simulink model "Quad_Nonlinear_Pitch_Model"  (R2020a)
settings: Solver=ode3  StartTime=0.0  StopTime=10  FixedStep=0.02  RelTol=1e-3
InitFcn:
  | LQR_Solver;
values from neighbouring files (symbols this model uses):
  B1 = (h_cg * g * m_tot) / (m_tot * h_cg^2 + J_yy)    [QuadConstants.m]    (also in pitch_parameter_estiation_result.m = 3.24098484589; pitch_parameter_estiation_result_II.m = 4.3602681386)
  B5 = (m2 * g * miu_k * r_y) / (m_tot * h_cg^2 + J_yy)    [QuadConstants.m]    (also in pitch_parameter_estiation_result.m = 0.171406679098; pitch_parameter_estiation_result_II.m = 0.59598011023)
undefined symbols (not defined in the file or in its folder): Ba, I, K
libraries: simulink x1, eeGeneralControl x1
settings Model: Creator=Ali  LastModifiedBy=Ali

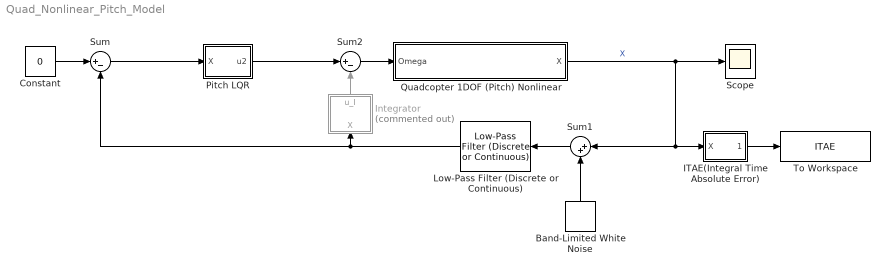
== system Quad_Nonlinear_Pitch_Model ==
  Band-Limited White Noise : simulink/Sources/Band-Limited White Noise  Cov=[0.0001]  Ts=0.02  seed=[23341]
  Constant : Constant  Value=0
  ITAE(Integral Time Absolute Error) : Subsystem
  Integrator : Subsystem  Commented=on
  Low-Pass Filter (Discrete or Continuous) : eeGeneralControl/Low-Pass Filter (Discrete or Continuous)  K=1  T=0.05  B=inf  A=-inf  init_option=Inherited from block input  x0=0  Ts=0
  Pitch LQR : Subsystem
  Quadcopter 1DOF (Pitch) Nonlinear : Subsystem  TreatAsAtomicUnit=on
      mask Display: image('Seesaw.png'); % Use "Edit Image" on toolstrip to change.
  Scope : Scope
  Sum : Sum  Inputs=|+-
  Sum1 : Sum  Inputs=|++
  Sum2 : Sum  Inputs=|+-
  To Workspace : ToWorkspace  VariableName=ITAE  SaveFormat=Timeseries  SampleTime=-1
  wires:
  Quadcopter 1DOF (Pitch) Nonlinear/1(X) -> Sum1/1, ITAE(Integral Time Absolute Error)/1(X), Scope/1  "X"
  Constant/1 -> Sum/1
  ITAE(Integral Time Absolute Error)/1(ITAE) -> To Workspace/1
  Band-Limited White Noise/1 -> Sum1/2
  Sum1/1 -> Low-Pass Filter (Discrete or Continuous)/1
  Pitch LQR/1(u2) -> Sum2/1
  Sum2/1 -> Quadcopter 1DOF (Pitch) Nonlinear/1(Omega)
  Integrator/1(u_I) -> Sum2/2
  Sum/1 -> Pitch LQR/1(X)
  Low-Pass Filter (Discrete or Continuous)/1 -> Integrator/1(X), Sum/2

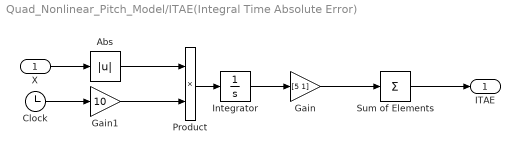
== system Quad_Nonlinear_Pitch_Model/ITAE(Integral Time Absolute Error) ==
  X : Inport
  Abs : Abs
  Clock : Clock
  Gain : Gain  Gain=[5 1]
  Gain1 : Gain  Gain=10
  Integrator : Integrator
  Product : Product
  Sum of Elements : Sum  Inputs=+
  ITAE : Outport
  wires:
  Product/1 -> Integrator/1
  Integrator/1 -> Gain/1
  Clock/1 -> Gain1/1
  Sum of Elements/1 -> ITAE/1
  Abs/1 -> Product/1
  X/1 -> Abs/1
  Gain/1 -> Sum of Elements/1
  Gain1/1 -> Product/2

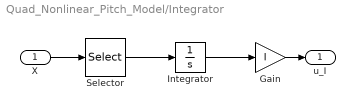
== system Quad_Nonlinear_Pitch_Model/Integrator ==
  X : Inport
  Gain : Gain  Gain=I
  Integrator : Integrator
  Selector : Selector  InputPortWidth=2  IndexOptions=Index vector (dialog)  Indices=[1]  OutputSizes=1
  u_I : Outport
  wires:
  Gain/1 -> u_I/1
  X/1 -> Selector/1
  Integrator/1 -> Gain/1
  Selector/1 -> Integrator/1

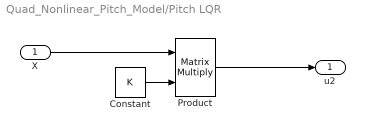
== system Quad_Nonlinear_Pitch_Model/Pitch LQR ==
  X : Inport
  Constant : Constant  Value=K
  Product : Product  Multiplication=Matrix(*)
  u2 : Outport
  wires:
  Product/1 -> u2/1
  Constant/1 -> Product/2
  X/1 -> Product/1

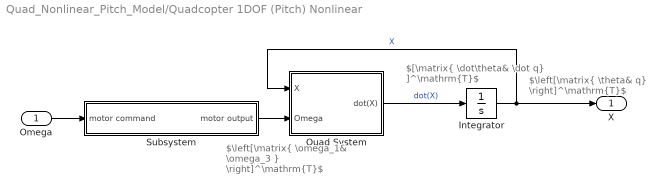
== system Quad_Nonlinear_Pitch_Model/Quadcopter 1DOF (Pitch) Nonlinear ==
  note: $\left[\matrix{ \omega_1& \omega_3 } \right]^\mathrm{T}$
  note: $\left[\matrix{ \theta& q} \right]^\mathrm{T}$
  note: $[\matrix{ \dot\theta& \dot q} ]^\mathrm{T}$
  Omega : Inport
  Integrator : Integrator  InitialCondition=[0.9628, 0]
  Quad System : Subsystem
  Subsystem : Subsystem
  X : Outport
  wires:
  Integrator/1 -> X/1, Quad System/1(X)  "X"
  Quad System/1(dot(X)) -> Integrator/1  "dot(X)"
  Omega/1 -> Subsystem/1(motor command)
  Subsystem/1(motor output) -> Quad System/2(Omega)

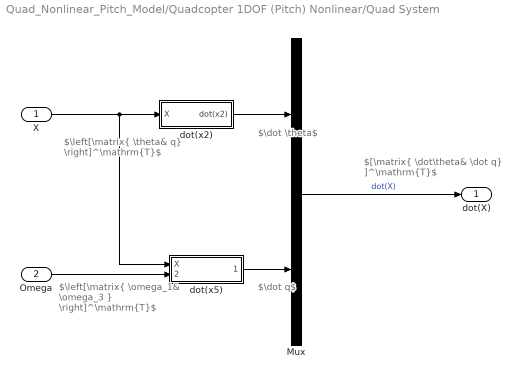
== system Quad_Nonlinear_Pitch_Model/Quadcopter 1DOF (Pitch) Nonlinear/Quad System ==
  note: $\dot \theta$
  note: $\left[\matrix{ \theta& q} \right]^\mathrm{T}$
  note: $[\matrix{ \dot\theta& \dot q} ]^\mathrm{T}$
  note: $\left[\matrix{ \omega_1& \omega_3 } \right]^\mathrm{T}$
  note: $\dot q$
  X : Inport
  Omega : Inport  Port=2
  Mux : Mux  Inputs=2
  dot(x2) : Subsystem
  dot(x5) : Subsystem
  dot(X) : Outport
  wires:
  Mux/1 -> dot(X)/1  "dot(X)"
  dot(x2)/1(dot(x2)) -> Mux/1
  dot(x5)/1(dot(x5)) -> Mux/2
  X/1 -> dot(x5)/1(X), dot(x2)/1(X)
  Omega/1 -> dot(x5)/2(Omega)

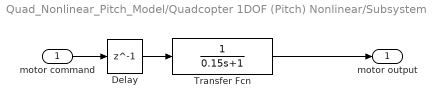
== system Quad_Nonlinear_Pitch_Model/Quadcopter 1DOF (Pitch) Nonlinear/Subsystem ==
  motor command : Inport
  Delay : Delay  DelayLength=1
  Transfer Fcn : TransferFcn  Denominator=[0.15 1]
  motor output : Outport
  wires:
  Transfer Fcn/1 -> motor output/1
  motor command/1 -> Delay/1
  Delay/1 -> Transfer Fcn/1

== system Quad_Nonlinear_Pitch_Model/Quadcopter 1DOF (Pitch) Nonlinear/Quad System/dot(x2) ==
  X : Inport
  1 : Subsystem
  dot(x2) : Outport
  wires:
  X/1 -> 1/1(X)  "X"
  1/1(x5cos(x1)) -> dot(x2)/1

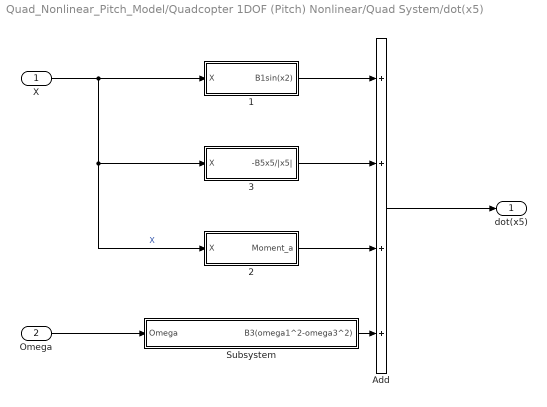
== system Quad_Nonlinear_Pitch_Model/Quadcopter 1DOF (Pitch) Nonlinear/Quad System/dot(x5) ==
  X : Inport
  Omega : Inport  Port=2
  1 : Subsystem
  2 : Subsystem
  3 : Subsystem
  Add : Sum  Inputs=++++
  Subsystem : Subsystem
  dot(x5) : Outport
  wires:
  X/1 -> 2/1(X), 3/1(X), 1/1(X)  "X"
  Omega/1 -> Subsystem/1(Omega)
  Add/1 -> dot(x5)/1
  3/1("-B5x5/|x5| ") -> Add/2
  1/1(B1sin(x2)) -> Add/1
  Subsystem/1(B3(omega1^2-omega3^2)) -> Add/4
  2/1(Moment_a) -> Add/3

== system Quad_Nonlinear_Pitch_Model/Quadcopter 1DOF (Pitch) Nonlinear/Quad System/dot(x2)/1 ==
  X : Inport
  Selector : Selector  InputPortWidth=2  IndexOptions=Index vector (dialog)  Indices=[2]  OutputSizes=1
  x5cos(x1) : Outport
  wires:
  X/1 -> Selector/1  "x"
  Selector/1 -> x5cos(x1)/1

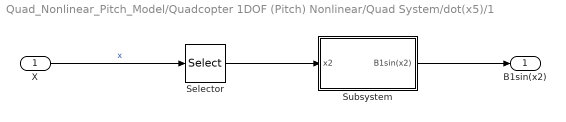
== system Quad_Nonlinear_Pitch_Model/Quadcopter 1DOF (Pitch) Nonlinear/Quad System/dot(x5)/1 ==
  X : Inport
  Selector : Selector  InputPortWidth=2  IndexOptions=Index vector (dialog)  Indices=[1]  OutputSizes=1
  Subsystem : Subsystem
  B1sin(x2) : Outport
  wires:
  X/1 -> Selector/1  "x"
  Subsystem/1(B1sin(x2)) -> B1sin(x2)/1
  Selector/1 -> Subsystem/1(x2)

== system Quad_Nonlinear_Pitch_Model/Quadcopter 1DOF (Pitch) Nonlinear/Quad System/dot(x5)/2 ==
  X : Inport
  Selector : Selector  InputPortWidth=2  IndexOptions=Index vector (dialog)  Indices=[1]  OutputSizes=1
  Subsystem : Subsystem
  Moment_a : Outport
  wires:
  X/1 -> Selector/1  "x"
  Subsystem/1(moment_a) -> Moment_a/1
  Selector/1 -> Subsystem/1(In1)

== system Quad_Nonlinear_Pitch_Model/Quadcopter 1DOF (Pitch) Nonlinear/Quad System/dot(x5)/3 ==
  X : Inport
  Selector : Selector  InputPortWidth=2  IndexOptions=Index vector (dialog)  Indices=[2]  OutputSizes=1
  Subsystem : Subsystem
  "-B5x5/|x5| " : Outport
  wires:
  X/1 -> Selector/1  "x"
  Subsystem/1("-B5x5/|x5| ") -> "-B5x5/|x5| "/1
  Selector/1 -> Subsystem/1(x5)

== system Quad_Nonlinear_Pitch_Model/Quadcopter 1DOF (Pitch) Nonlinear/Quad System/dot(x5)/Subsystem ==
  Omega : Inport
  B3(omega1^2-omega3^2) : Outport
  wires:
  Omega/1 -> B3(omega1^2-omega3^2)/1

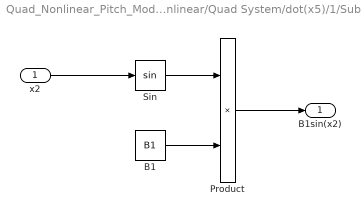
== system Quad_Nonlinear_Pitch_Model/Quadcopter 1DOF (Pitch) Nonlinear/Quad System/dot(x5)/1/Subsystem ==
  x2 : Inport
  B1 : Constant  Value=B1
  Product : Product
  Sin : Trigonometry
  B1sin(x2) : Outport
  wires:
  Product/1 -> B1sin(x2)/1
  x2/1 -> Sin/1
  B1/1 -> Product/2
  Sin/1 -> Product/1

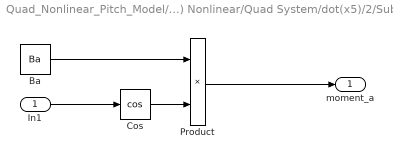
== system Quad_Nonlinear_Pitch_Model/Quadcopter 1DOF (Pitch) Nonlinear/Quad System/dot(x5)/2/Subsystem ==
  In1 : Inport
  Ba : Constant  Value=Ba
  Cos : Trigonometry  Operator=cos
  Product : Product
  moment_a : Outport
  wires:
  Product/1 -> moment_a/1
  Ba/1 -> Product/1
  In1/1 -> Cos/1
  Cos/1 -> Product/2

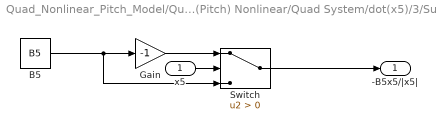
== system Quad_Nonlinear_Pitch_Model/Quadcopter 1DOF (Pitch) Nonlinear/Quad System/dot(x5)/3/Subsystem ==
  x5 : Inport
  B5 : Constant  Value=B5
  Gain : Gain  Gain=-1
  Switch : Switch  Criteria=u2 > Threshold
  "-B5x5/|x5| " : Outport
  wires:
  Switch/1 -> "-B5x5/|x5| "/1
  B5/1 -> Switch/3, Gain/1
  x5/1 -> Switch/2
  Gain/1 -> Switch/1
